simulink library "FaultManagement_lib"  (R2022b)
settings: Solver=VariableStepAuto  StartTime=0.0  StopTime=10.0  RelTol=1e-3
undefined symbols (not defined in the file or in its folder): Fault1, FaultName
settings Model: Creator=cpatel  LastModifiedBy=cpatel
settings ModelReferenceCC: EnableRefExpFcnMdlSchedulingChecks=on

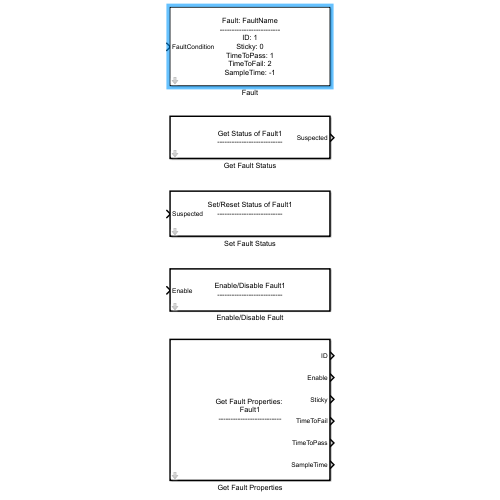
[thumbnail: Simulink's stored preview of the top-level diagram]
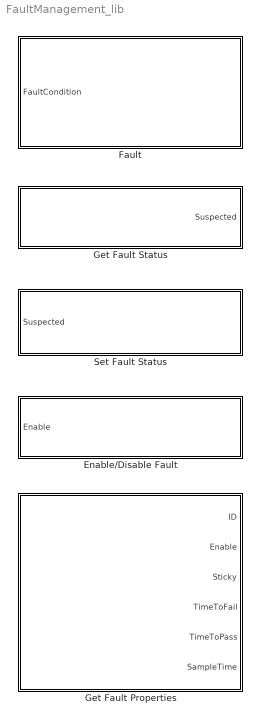
== system FaultManagement_lib ==
  Enable/Disable Fault : Subsystem  TreatAsAtomicUnit=on  mask{FaultName=Fault1}
      mask prompts: FaultName "Select Fault:"
      mask Callback FaultName:
      | fltName = get_param(gcb,'FaultName');
      | 
      |     % Update Data Store Write Block
      |     dsWrtBlkHdl = find_system(gcb,'SearchDepth',1,'LookUnderMasks','on','FollowLinks','on','BlockType','DataStoreWrite');
      |     set_param(dsWrtBlkHdl{1},'DataStoreName',fltName,'DataStoreElements',[fltName,'.Enable']);
      mask DialogControl DescGroupVar Prompt: Enable/Disable Fault
      mask DialogControl DescTextVar Prompt: Use this block to enable or disable selected fault.
      mask DialogControl ParameterGroupVar Prompt: Select fault event from the list
      mask Display:
      | disp(['Enable/Disable ', get_param(gcb,'FaultName'),newline, ...
      |     '---------------------------']);
  Fault : Subsystem  mask(Fault Block){FaultName=FaultName, ID=1, Enable=1, Sticky=0, TimeToFail=1, TimeToPass=2, SampleTime=-1}
      mask prompts: FaultName "Select Fault:"; ID "Fault ID (uint16):"; Enable "Fault Enable (Boolean):"; Sticky "Fault Type (Sticky/Non-Sticky):"; TimeToFail "Fault Time To Fail (Seconds):"; TimeToPass "Fault Time To Pass (Seconds):"; SampleTime "Fault Sample Time"
      mask help: Fault block implements fault maturity logic and updates fault status (Suspected, Active and Occured) based on FaultCondition input.
      settings: LibrarySourceBlock=FaultManagement_lib/Fault
      mask Callback FaultName:
      | fltName = get_param(gcb,'FaultName');
      |     temp = split(gcs,'/');
      |     mdlName = temp{1};
      |     if isequal(get_param(mdlName,'BlockDiagramType'),'library')
      |         id = uint16(1);
      |         enable = true;
      |         sticky = false;
      |         timeToFail = single(1);
      |         timeToPass = single(2);
      |         sampleTime = -1;
      |     else
      |         a = Simulink.data.evalinGlobal(mdlName,['FaultInit.',fltName]);
      |         id = a.ID;
      |         enable = a.Enable;
      |         sticky = a.Sticky;
      |         timeToFail = a.TimeToFail;
      |         timeToPass = a.TimeToPass;
      |         sampleTime = a.SampleTime;
      |     end
      |         % Data Store Write Block
      |         dsWrtBlkHdl = find_system(gcb,'SearchDepth',1,'LookUnderMasks','on','FollowLinks','on','BlockType','DataStoreWrite');
      |         ElementList = [fltName,'.Suspected#',fltName,'.Active#',fltName,'.Occured'];
      |         set_param(dsWrtBlkHdl{1},'DataStoreName',fltName,'DataStoreElements',ElementList);
      | 
      |         % Data Store Read Block
      |         dsRdBlkHdl = find_system(gcb,'SearchDepth',1,'LookUnderMasks','on','FollowLinks','on','BlockType','DataStoreRead');
      |         ElementList = [fltName,'.Enable#',fltName,'.Sticky#',fltName,'.TimeToFail#', fltName,'.TimeToPass#',fltName,'.SampleTime'];
      |         set_param(dsRdBlkHdl{1},'DataStoreName',fltName,'DataStoreElements',ElementList);
      | 
      |         % Input Sample Time
      |         inPortBlkHdl = find_system(gcb,'SearchDepth',1,'LookUnderMasks','on','FollowLinks','on','BlockType','Inport');
      |         for i = 1:length(inPortBlkHdl)
      |             set_param(inPortBlkHdl{i},'SampleTime',num2str(sampleTime));
      |         end
      | 
      |         % Update Block Parameters
      |         set_param(gcb,'FaultName',fltName);
      |         set_param(gcb,'ID',num2str(id));
      |         set_param(gcb,'Enable',num2str(enable));
      |         set_param(gcb,'Sticky',num2str(sticky));
      |         set_param(gcb,'TimeToFail',num2str(timeToFail));
      |         set_param(gcb,'TimeToPass',num2str(timeToPass));
      |         set_param(gcb,'SampleTime', num2str(sampleTime));
      mask Display:
      | disp(['Fault: ', get_param(gcb,'FaultName'),newline, ...
      |     '-------------------------', newline, ...
      |     'ID: ', get_param(gcb,'ID'), newline, ...
      |     'Sticky: ', get_param(gcb,'Sticky'), newline, ...
      |     'TimeToPass: ', get_param(gcb,'TimeToFail'), newline, ...
      |     'TimeToFail: ', get_param(gcb,'TimeToPass'), newline, ...
      |     'SampleTime: ', get_param(gcb,'SampleTime') ...
      |     ]);
  Get Fault Properties : Subsystem  TreatAsAtomicUnit=on  mask{FaultName=Fault1}
      mask prompts: FaultName "Select Fault:"
      mask Callback FaultName:
      | fltName = get_param(gcb,'FaultName');
      |     % Update Data Store Read Block Parameters
      |     set_param(gcb,'FaultName',fltName);
      |     dsRdBlkHdl = find_system(gcb,'SearchDepth',1,'LookUnderMasks','on','FollowLinks','on','BlockType','DataStoreRead');
      |     set_param(dsRdBlkHdl{1},'DataStoreName',fltName,...
      |         'DataStoreElements',[fltName,'.ID#', fltName,'.Enable#', ...
      |                             fltName,'.Sticky#', fltName,'.TimeToFail#',...
      |                             fltName,'.TimeToPass#', fltName,'.SampleTime']);
      mask DialogControl DescGroupVar Prompt: Get Fault Properties
      mask DialogControl DescTextVar Prompt: Get properties of a selected Fault Event.
      mask DialogControl ParameterGroupVar Prompt: Select fault event from the list
      mask Display:
      | disp(['Get Fault Properties: ', newline, ...
      |     get_param(gcb,'FaultName'), newline, ...
      |     '--------------------------']);
  Get Fault Status : Subsystem  TreatAsAtomicUnit=on  mask{FaultName=Fault1, StatusField=Suspected}
      mask prompts: FaultName "Select Fault:"; StatusField "Select Fault Status Field:"
      mask Callback FaultName:
      | fltName = get_param(gcb,'FaultName');
      |     fltStatus = get_param(gcb,'StatusField');
      |     dsRdBlkHdl = find_system(gcb,'SearchDepth',1,'LookUnderMasks','on','FollowLinks','on','BlockType','DataStoreRead');
      |     set_param(dsRdBlkHdl{1},'DataStoreName',fltName,...
      |         'DataStoreElements',[fltName,'.',fltStatus]);
      mask TypeOptions StatusField: Suspected | Active | Occured
      mask Callback StatusField:
      | fltName = get_param(gcb,'FaultName');
      |     fltStatus = get_param(gcb,'StatusField');
      | 
      |     % Update Data Store:
      |     dsRdBlkHdl = find_system(gcb,'SearchDepth',1,'LookUnderMasks','on', ...
      |         'FollowLinks','on','BlockType','DataStoreRead');
      |     set_param(dsRdBlkHdl{1},'DataStoreName',fltName,'DataStoreElements',[fltName,'.',fltStatus]);
      | 
      |     % Update Name of Inport
      |     outBlgHdl = find_system(gcb,'SearchDepth',1,'LookUnderMasks','on', ...
      |         'FollowLinks','on','BlockType','Outport');
      |     set_param(outBlgHdl{1},'Name',fltStatus);
      mask DialogControl DescGroupVar Prompt: Get Fault State
      mask DialogControl DescTextVar Prompt: Get state of a selected Fault Event.
      mask DialogControl ParameterGroupVar Prompt: Select Fault event from the list
      mask Display:
      | disp(['Get Status of ', get_param(gcb,'FaultName'),newline, ...
      |     '---------------------------']);
  Set Fault Status : Subsystem  TreatAsAtomicUnit=on  mask{StatusField=Suspected, FaultName=Fault1}
      mask prompts: StatusField "Select Fault Status Field:"; FaultName "Select Fault:"
      mask TypeOptions StatusField: Suspected | Active | Occured
      mask Callback StatusField:
      | fltName = get_param(gcb,'FaultName');
      |     fltStatus = get_param(gcb,'StatusField');
      | 
      |     % Update Data Store:
      |     dsWrtBlkHdl = find_system(gcb,'SearchDepth',1,'LookUnderMasks','on', ...
      |         'FollowLinks','on','BlockType','DataStoreWrite');
      |     set_param(dsWrtBlkHdl{1},'DataStoreName',fltName,'DataStoreElements',[fltName,'.',fltStatus]);
      | 
      |     % Update Name of Inport
      |     inBlgHdl = find_system(gcb,'SearchDepth',1,'LookUnderMasks','on', ...
      |         'FollowLinks','on','BlockType','Inport');
      |     set_param(inBlgHdl{1},'Name',fltStatus);
      mask Callback FaultName:
      | fltName = get_param(gcb,'FaultName');
      |     fltStatus = get_param(gcb,'StatusField');
      | 
      |     dsWrtBlkHdl = find_system(gcb,'SearchDepth',1,'LookUnderMasks','on','FollowLinks','on','BlockType','DataStoreWrite');
      |     set_param(dsWrtBlkHdl{1},'DataStoreName',fltName,...
      |         'DataStoreElements',[fltName,'.',fltStatus]);
      mask DialogControl DescGroupVar Prompt: Set Fault Status
      mask DialogControl DescTextVar Prompt: This block sets the status of a selected fault.
      mask DialogControl ParameterGroupVar Prompt: Select fault event from the list
      mask Display:
      | disp(['Set/Reset Status of ', ...
      |     get_param(gcb,'FaultName'),newline, ...
      |     '---------------------------', newline, ...
      |     ]);

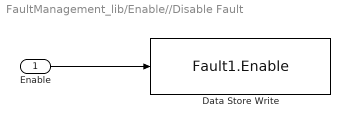
== system FaultManagement_lib/Enable//Disable Fault ==
  Enable : Inport
  Data Store Write : DataStoreWrite  DataStoreName=Fault1  DataStoreElements=Fault1.Enable  IndexOptions=Index vector (dialog)  Indices=1  OutputSizes=1
  wires:
  Enable/1 -> Data Store Write/1

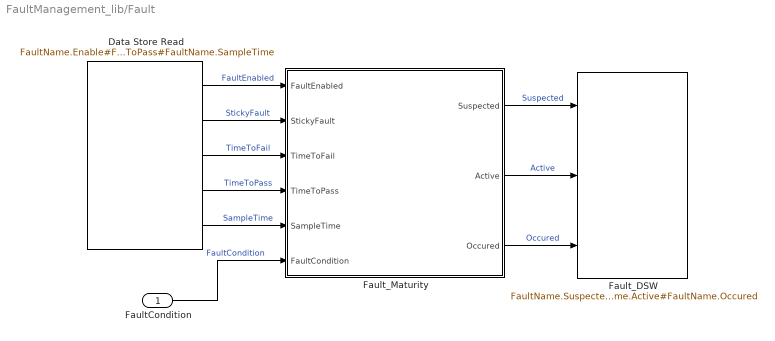
== system FaultManagement_lib/Fault ==
  FaultCondition : Inport
  Data Store Read : DataStoreRead  DataStoreName=FaultName  DataStoreElements=FaultName.Enable#FaultName.Sticky#FaultName.TimeToFail#FaultName.TimeToPass#FaultName.SampleTime  IndexOptions=Index vector (dialog)  Indices=1  OutputSizes=1
  Fault_DSW : DataStoreWrite  DataStoreName=FaultName  DataStoreElements=FaultName.Suspected#FaultName.Active#FaultName.Occured  IndexOptions=Starting index (dialog)  Indices=2  OutputSizes=1
  Fault_Maturity : Stateflow chart  TreatAsAtomicUnit=on
      settings: RTWSystemCode=Inline
  wires:
  Fault_Maturity/3(" Occured") -> Fault_DSW/3  "Occured"
  Fault_Maturity/2(" Active") -> Fault_DSW/2  "Active"
  Fault_Maturity/1(" Suspected") -> Fault_DSW/1  "Suspected"
  Data Store Read/4 -> Fault_Maturity/4(TimeToPass)  "TimeToPass"
  Data Store Read/3 -> Fault_Maturity/3(TimeToFail)  "TimeToFail"
  Data Store Read/2 -> Fault_Maturity/2(StickyFault)  "StickyFault"
  Data Store Read/5 -> Fault_Maturity/5(SampleTime)  "SampleTime"
  FaultCondition/1 -> Fault_Maturity/6(FaultCondition)  "FaultCondition"
  Data Store Read/1 -> Fault_Maturity/1(FaultEnabled)  "FaultEnabled"

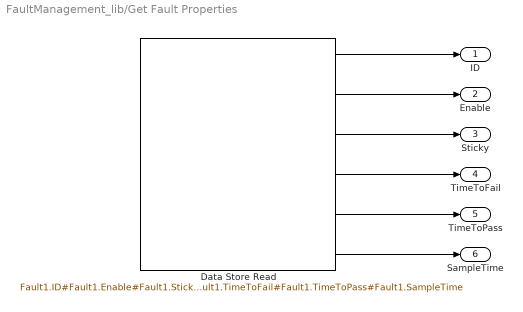
== system FaultManagement_lib/Get Fault Properties ==
  Data Store Read : DataStoreRead  DataStoreName=Fault1  DataStoreElements=Fault1.ID#Fault1.Enable#Fault1.Sticky#Fault1.TimeToFail#Fault1.TimeToPass#Fault1.SampleTime  IndexOptions=Index vector (dialog)  Indices=1  OutputSizes=1
  ID : Outport
  Enable : Outport  Port=2
  Sticky : Outport  Port=3
  TimeToFail : Outport  Port=4
  TimeToPass : Outport  Port=5
  SampleTime : Outport  Port=6
  wires:
  Data Store Read/1 -> ID/1
  Data Store Read/2 -> Enable/1
  Data Store Read/3 -> Sticky/1
  Data Store Read/4 -> TimeToFail/1
  Data Store Read/5 -> TimeToPass/1
  Data Store Read/6 -> SampleTime/1

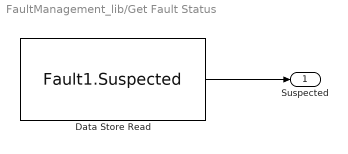
== system FaultManagement_lib/Get Fault Status ==
  Data Store Read : DataStoreRead  DataStoreName=Fault1  DataStoreElements=Fault1.Suspected  IndexOptions=Index vector (dialog)  Indices=1  OutputSizes=1
  Suspected : Outport
  wires:
  Data Store Read/1 -> Suspected/1

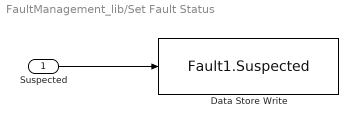
== system FaultManagement_lib/Set Fault Status ==
  Suspected : Inport
  Data Store Write : DataStoreWrite  DataStoreName=Fault1  DataStoreElements=Fault1.Suspected  IndexOptions=Index vector (dialog)  Indices=1  OutputSizes=1
  wires:
  Suspected/1 -> Data Store Write/1

== stateflow chart FaultManagement_lib/Fault/Fault_Maturity ==
  state Suspected_State [parallel]
    settings: executionOrder=1
    state NotSuspected
      if FaultEnabled
      if Index <= single(0)
      Test_Passed = true;
      Test_Failed = false;
      Index = single(0);
      else
      Index = max(single(0), Index - DwnCount);
      end
      else
      Index = single(0);
      Test_Passed = false;
      Test_Failed = false;
      end
    state Suspected
      if Index >= single(1)
      Test_Failed = true;
      Test_Passed = false;
      Index = single(1);
      else
      Index = min(single(1), Index + UpCount);
      end
    (default) -> NotSuspected : {DwnCount = SampleTime/TimeToPass;
        | UpCount = SampleTime/TimeToFail;}
    NotSuspected -> Suspected : [FaultCondition && FaultEnabled]
    Suspected -> NotSuspected [order 1] : [~FaultEnabled]{Index = single(0);}
    Suspected -> NotSuspected [order 2] : [~FaultCondition]
  state Active_State [parallel]
    settings: executionOrder=2
    state Inactive
    state Active
    (default) -> Inactive
    Inactive -> Active : [Test_Failed]
    Active -> Inactive [order 1] : [~FaultEnabled]
    Active -> Inactive [order 2] : [Test_Passed && ~StickyFault]{Fault_Occured = true;}
  state Occured_State [parallel]
    settings: executionOrder=3
    state NotOccured
      Fault_Occured = false;
    state Occured
    (default) -> NotOccured
    NotOccured -> Occured : [Fault_Occured]
    Occured -> NotOccured : [~FaultEnabled]
  data: FaultEnabled input; StickyFault input boolean; TimeToFail input single; Index local single size=1 =single(0); DwnCount local; UpCount local; TimeToPass input; SampleTime input; FaultCondition input; Suspected output boolean; Active output boolean; Occured output boolean; Test_Passed local =false; Test_Failed local =false; Fault_Occured local =false
